simulink library "INT_APP_SelSig"  (R2016b)
settings: Solver=VariableStepAuto  StartTime=0.0  StopTime=10.0  RelTol=1e-3
settings Model: Creator=bianxuyin  LastModifiedBy=bianxuyin

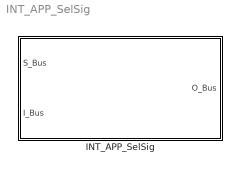
== system INT_APP_SelSig ==
  INT_APP_SelSig : Subsystem

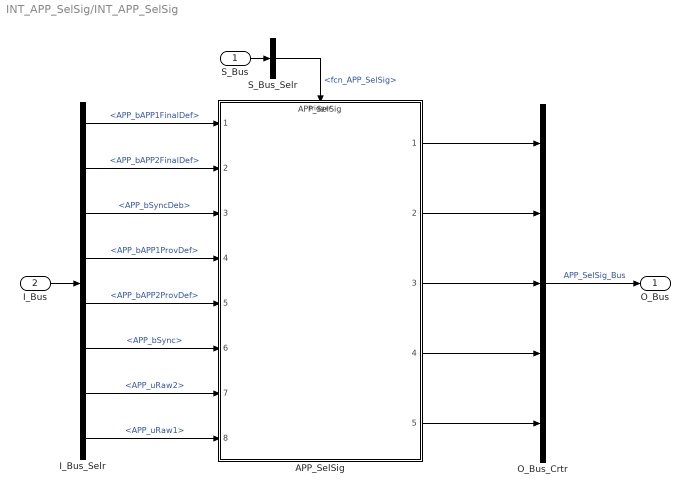
== system INT_APP_SelSig/INT_APP_SelSig ==
  S_Bus : Inport
  I_Bus : Inport  Port=2
  APP_SelSig : ModelReference  ModelNameDialog=APP_SelSig  SimulationMode=Normal  ModelReferenceVersion=1.26  TriggerPortName=function  TriggerPortTriggerType=function-call  TriggerPortStatesWhenEnabling=held
  I_Bus_Selr : BusSelector  OutputSignals=APP_bAPP1FinalDef,APP_bAPP2FinalDef,APP_bSyncDeb,APP_bAPP1ProvDef,APP_bAPP2ProvDef,APP_bSync,APP_uRaw2,APP_uRaw1
  O_Bus_Crtr : BusCreator  Inputs=5
  S_Bus_Selr : BusSelector  OutputSignals=fcn_APP_SelSig
  O_Bus : Outport
  wires:
  S_Bus_Selr/1 -> APP_SelSig/Trigger  "<fcn_APP_SelSig>"
  S_Bus/1 -> S_Bus_Selr/1
  I_Bus/1 -> I_Bus_Selr/1
  I_Bus_Selr/1 -> APP_SelSig/1  "<APP_bAPP1FinalDef>"
  I_Bus_Selr/2 -> APP_SelSig/2  "<APP_bAPP2FinalDef>"
  I_Bus_Selr/3 -> APP_SelSig/3  "<APP_bSyncDeb>"
  I_Bus_Selr/4 -> APP_SelSig/4  "<APP_bAPP1ProvDef>"
  I_Bus_Selr/5 -> APP_SelSig/5  "<APP_bAPP2ProvDef>"
  I_Bus_Selr/6 -> APP_SelSig/6  "<APP_bSync>"
  I_Bus_Selr/7 -> APP_SelSig/7  "<APP_uRaw2>"
  I_Bus_Selr/8 -> APP_SelSig/8  "<APP_uRaw1>"
  O_Bus_Crtr/1 -> O_Bus/1  "APP_SelSig_Bus"
  APP_SelSig/1 -> O_Bus_Crtr/1
  APP_SelSig/2 -> O_Bus_Crtr/2
  APP_SelSig/3 -> O_Bus_Crtr/3
  APP_SelSig/4 -> O_Bus_Crtr/4
  APP_SelSig/5 -> O_Bus_Crtr/5
